simulink model "decoder"  (R2013b)
settings: Solver=FixedStepDiscrete  StartTime=0.0  StopTime=300  FixedStep=1  RelTol=1e-3
settings Model: Creator=qiji  LastModifiedBy=qiji
settings OptimizationCC: BlockReduction=off  ConditionallyExecuteInputs=off
settings DebuggingCC: SingleTaskRateTransMsg=error

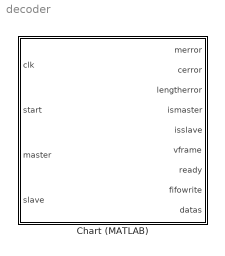
== system decoder ==
  Chart (MATLAB) : Stateflow chart  TreatAsAtomicUnit=on

== stateflow chart decoder/Chart (MATLAB) ==
  state s000
    en:
    masterframe=false;
    slaveframe<=false;
    sample8<=[false; false; false];
    du:
    checkcode=[false; false; false; false;...
    false; false; false; false];
    dataRegisters=[false; false; false; false;...
    false; false; false; false;...
    false; false; false; false;...
    false; false; false; false;];
    samples = [false; false; false; false];
    total=[false; false; false];
    counter8=[false; false; false];
    merror=false;
    cerror=false;
    ismaster=false;
    isslave=false;
    ready=false;
    fifowrite=false;
    datas=[false; false; false; false;...
    false; false; false; false;...
    false; false; false; false;...
    false; false; false; false;];;
    prostate=[false; false];
    cerrorflag=false;
    cfl=[false; false; false; false; false];
    overflow=false;
    lengtherror=false;
    vframe=false;
  state s001
  state s100
  state s101
  state s010
  state s011
  s100 -> s101 : [sample8(1)==true && sample8(2)==true...
      | && sample8(3)==true]
  s000 -> s001 : [start == true]
      | {
      | masterframe=master;
      | slaveframe=slave;
      | sample8=[true; false; false];
      | state=[false; false; false];
      | }
  s001 -> s010 : [sample8(1)==true && sample8(2)==true...
      | && sample8(3)==true]
  s011 -> s100 : [sample8(1)==true && sample8(2)==true...
      | && sample8(3)==true]
  (default) -> s000
  s010 -> s011 : [sample8(1)==true && sample8(2)==true...
      | && sample8(3)==true]
  data: merror output boolean; cerror output boolean; lengtherror output boolean; ismaster output boolean; isslave output boolean; vframe output boolean; ready output boolean; fifowrite output boolean; datas output boolean size=16; checkcode local boolean size=8; dataRegisters local boolean size=16; masterframe local boolean; slaveframe local boolean; samples local boolean size=4; prostate local boolean size=2; total local boolean size=3; counter8 local boolean size=3; sample8 local boolean size=3; state local boolean size=3; cerrorflag local boolean; overflow local boolean; cfl local boolean size=5; clk input boolean; start input boolean; master input boolean; slave input boolean
  data checkcode settings: description=存放checkcode
  data dataRegisters settings: description=存放manchester解码后的数据
  data masterframe settings: description=the symbol of master frame
  data slaveframe settings: description=the symbol of slave frame
  data samples settings: description=store 4 bits sample value
  data prostate settings: description="current frame  length 帧长度计数器"
  data total settings: description=add 1 per 16 bit
  data counter8 settings: description=the number of data in dataRegisters
  data sample8 settings: description=sample the value per 8 cycle
  data state settings: description=the state of sampling data value
  data cerrorflag settings: description=标识符：标识校验码错误；‘1’表示有校验码错误，‘0’表示没有检验码错误
  data overflow settings: description=溢出标识位：‘1’表示有溢出，‘0’表示没有溢出
